simulink model "odom_waypoint"  (R2022a)
settings: Solver=FixedStepDiscrete  StartTime=0.0  StopTime=inf  FixedStep=0.05  RelTol=1e-3  EnableMultiTasking=on
undefined symbols (not defined in the file): Angular, Linear
libraries: robotlib x4
settings Model: Creator=The MathWorks, Inc.  LastModifiedBy=lcrist
settings SolverCC: AlgebraicLoopSolver=TrustRegion
settings DataIOCC: LimitDataPoints=on  SaveFormat=Array  ReturnWorkspaceOutputs=off
settings OptimizationCC: DefaultUnderspecifiedDataType=single  ZeroExternalMemoryAtStartup=off  ZeroInternalMemoryAtStartup=off  LifeSpan=1  MaxStackSize=64
settings DebuggingCC: SolverPrmCheckMsg=warning  UnconnectedInputMsg=warning  UnconnectedOutputMsg=warning  UnconnectedLineMsg=warning  SFUnexpectedBacktrackingDiag=warning  SFNoUnconditionalDefaultTransitionDiag=warning  SFExecutionAtInitializationDiag=none  SFMachineParentedDataDiag=warning  ArithmeticOperatorsInVariantConditions=warning
settings HardwareCC: ProdBitPerPointer=32  ProdBitPerSizeT=32  ProdBitPerPtrDiffT=32  ProdLargestAtomicFloat=None  ProdIntDivRoundTo=Undefined  ProdEndianess=Unspecified  ProdWordSize=32  ProdHWDeviceType=Generic->Unspecified (assume 32-bit Generic)  TargetHWDeviceType=Generic->Unspecified (assume 32-bit Generic)  UseEmbeddedCoderFeatures=off
settings ModelReferenceCC: PropagateSignalLabelsOutOfModel=off
settings SFSimCC: SimUseLocalCustomCode=off  CustomCodeUndefinedFunction=UseInterfaceOnly  SimTargetLang=C++
settings RTWCC: SystemTargetFile=ert.tlc  HardwareBoard=Robot Operating System (ROS)  TLCOptions=-aInlineSetEventsForThisBaseRateFcn=TLC_FALSE -aSuppressMultiTaskScheduler=TLC_FALSE -aRateBasedStepFcn=0  TemplateMakefile=ert_default_tmf  RTWUseLocalCustomCode=off  Toolchain=Catkin  TargetLang=C++
settings CodeAppCC: StateflowObjectComments=on
settings ERTTargetCC: MultiwordLength=2048  ERTCustomFileBanners=off  CodeInterfacePackaging=C++ class  SupportContinuousTime=on  SupportNonInlinedSFcns=on  RemoveResetFunc=off  SupportVariableSizeSignals=on  ModelStepFunctionPrototypeControlCompliant=off  RootIOFormat=Structure reference  ConvertIfToSwitch=off  SuppressUnreachableDefaultCases=off
settings ConfigComp: CovMetricSettings=dw  CovSaveCumulativeToWorkspaceVar=on  CovSaveSingleToWorkspaceVar=on  CovExternalEMLEnable=off  CovSFcnEnable=off

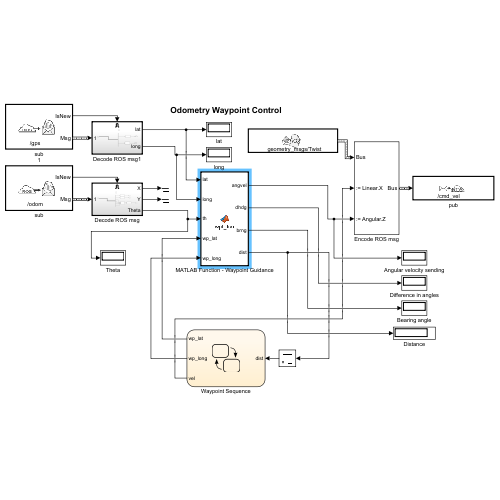
[thumbnail: Simulink's stored preview of the top-level diagram]
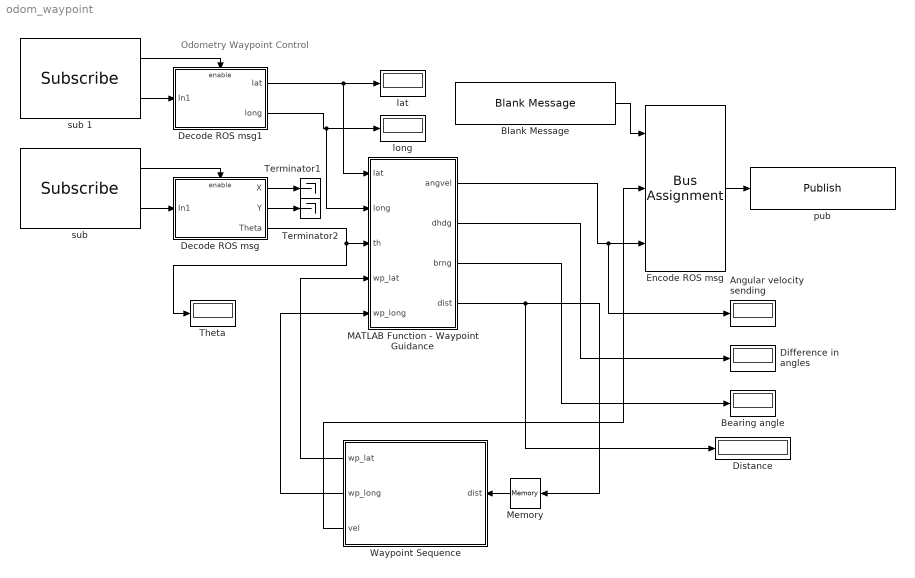
== system odom_waypoint ==
  note: Odometry Waypoint Control
  Angular velocity sending : Display
  Bearing angle : Display
  Blank Message : robotlib/Blank Message  messageClass=Message  entityType=geometry_msgs/Twist  messageType=geometry_msgs/Twist  SampleTime=inf  legacyBusStruct=off
  Decode ROS msg : Subsystem
  Decode ROS msg1 : Subsystem
  Difference in angles : Display
  Distance : Display
  Encode ROS msg : BusAssignment  AssignedSignals=Linear.X,Angular.Z
  MATLAB Function - Waypoint Guidance : MATLAB Function  TreatAsAtomicUnit=on
  Memory : Memory  InitialCondition=1
  Terminator1 : Terminator
  Terminator2 : Terminator
  Theta : Display
  Waypoint Sequence : Stateflow chart  TreatAsAtomicUnit=on
  lat : Display
  long : Display
  pub : robotlib/Publish  topicSource=Specify your own  topic=/cmd_vel  messageType=geometry_msgs/Twist  legacyBusStruct=off  messageQueueLength=105
  "sub " : robotlib/Subscribe  topicSource=Specify your own  topic=/odom  messageType=nav_msgs/Odometry  SampleTime=-1  legacyBusStruct=off  messageQueueLength=51
  sub 1 : robotlib/Subscribe  topicSource=Specify your own  topic=/gps  messageType=sensor_msgs/NavSatFix  SampleTime=-1  legacyBusStruct=off  messageQueueLength=51
  wires:
  Encode ROS msg/1 -> pub/1
  "sub "/1 -> Decode ROS msg/Enable
  "sub "/2 -> Decode ROS msg/1(In1)
  Blank Message/1 -> Encode ROS msg/1
  Decode ROS msg/3(Theta) -> MATLAB Function - Waypoint Guidance/3(th), Theta/1
  MATLAB Function - Waypoint Guidance/1(angvel) -> Encode ROS msg/3, Angular velocity sending/1
  Waypoint Sequence/1(wp_lat) -> MATLAB Function - Waypoint Guidance/4(wp_lat)
  Waypoint Sequence/2(wp_long) -> MATLAB Function - Waypoint Guidance/5(wp_long)
  Memory/1 -> Waypoint Sequence/1(dist)
  sub 1/2 -> Decode ROS msg1/1(In1)
  sub 1/1 -> Decode ROS msg1/Enable
  Decode ROS msg/1(X) -> Terminator1/1
  Decode ROS msg/2(Y) -> Terminator2/1
  Decode ROS msg1/1(lat) -> MATLAB Function - Waypoint Guidance/1(lat), lat/1
  Decode ROS msg1/2(long) -> MATLAB Function - Waypoint Guidance/2(long), long/1
  MATLAB Function - Waypoint Guidance/2(dhdg) -> Difference in angles/1
  MATLAB Function - Waypoint Guidance/3(brng) -> Bearing angle/1
  MATLAB Function - Waypoint Guidance/4(dist) -> Memory/1, Distance/1
  Waypoint Sequence/3(vel) -> Encode ROS msg/2

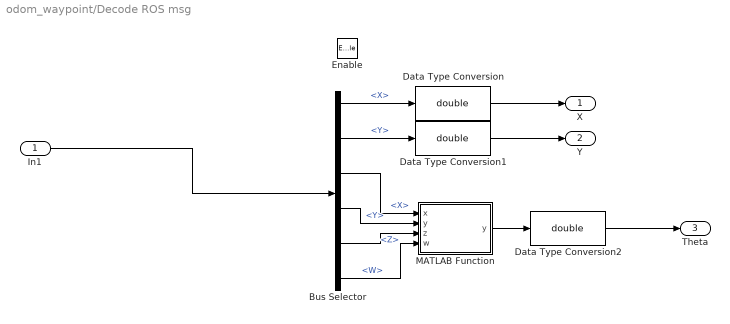
== system odom_waypoint/Decode ROS msg ==
  In1 : Inport
  Enable : EnablePort
  Bus Selector : BusSelector  DialogController=Simulink.DDGSource_BusSelector  OutputSignals=Pose.Pose.Position.X,Pose.Pose.Position.Y,Pose.Pose.Orientation.X,Pose.Pose.Orientation.Y,Pose.Pose.Orientation.Z,Pose.Pose.Orientation.W
  Data Type Conversion : DataTypeConversion  OutDataTypeStr=double  SaturateOnIntegerOverflow=off  RndMeth=Floor
  Data Type Conversion1 : DataTypeConversion  OutDataTypeStr=double  SaturateOnIntegerOverflow=off  RndMeth=Floor
  Data Type Conversion2 : DataTypeConversion  OutDataTypeStr=double  SaturateOnIntegerOverflow=off  RndMeth=Floor
  MATLAB Function : MATLAB Function  TreatAsAtomicUnit=on
  X : Outport  VectorParamsAs1DForOutWhenUnconnected=off
  Y : Outport  Port=2  VectorParamsAs1DForOutWhenUnconnected=off
  Theta : Outport  Port=3  VectorParamsAs1DForOutWhenUnconnected=off
  wires:
  In1/1 -> Bus Selector/1
  Bus Selector/2 -> Data Type Conversion1/1  "<Y>"
  Bus Selector/1 -> Data Type Conversion/1  "<X>"
  Data Type Conversion/1 -> X/1
  Data Type Conversion1/1 -> Y/1
  Data Type Conversion2/1 -> Theta/1
  MATLAB Function/1(y) -> Data Type Conversion2/1
  Bus Selector/3 -> MATLAB Function/1(x)  "<X>"
  Bus Selector/4 -> MATLAB Function/2("y ")  "<Y>"
  Bus Selector/5 -> MATLAB Function/3(z)  "<Z>"
  Bus Selector/6 -> MATLAB Function/4(w)  "<W>"

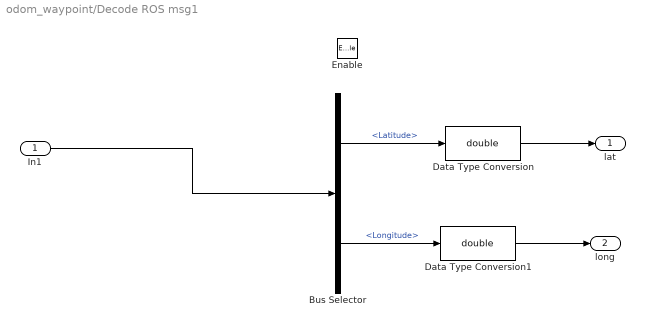
== system odom_waypoint/Decode ROS msg1 ==
  In1 : Inport
  Enable : EnablePort
  Bus Selector : BusSelector  DialogController=Simulink.DDGSource_BusSelector  OutputSignals=Latitude,Longitude
  Data Type Conversion : DataTypeConversion  OutDataTypeStr=double  SaturateOnIntegerOverflow=off  RndMeth=Floor
  Data Type Conversion1 : DataTypeConversion  OutDataTypeStr=double  SaturateOnIntegerOverflow=off  RndMeth=Floor
  lat : Outport  VectorParamsAs1DForOutWhenUnconnected=off
  long : Outport  Port=2  VectorParamsAs1DForOutWhenUnconnected=off
  wires:
  In1/1 -> Bus Selector/1
  Bus Selector/2 -> Data Type Conversion1/1  "<Longitude>"
  Bus Selector/1 -> Data Type Conversion/1  "<Latitude>"
  Data Type Conversion/1 -> lat/1
  Data Type Conversion1/1 -> long/1

== matlab function odom_waypoint/Decode ROS msg/MATLAB Function ==
  data: x input; y output; y input; z input; w input
function y = fcn(x,y,z,w)

eulZYX = quat2eul([x,y,z,w]);

y = eulZYX(3);

== matlab function odom_waypoint/MATLAB Function - Waypoint Guidance ==
  data: angvel output; lat input; long input; th input; wp_lat input; wp_long input; dhdg output; brng output; dist output
function [angvel, dhdg, brng, dist]  = wpt_fcn(lat,long,th,wp_lat,wp_long)
% Function to implement waypoint guidance
% Inputs:
%  - lat: Current lattitude position
%  - long: Current longitude position
%  - th: Current theta position
%  - wp_lat: Current waypoint goals, lattitude
%  - wp_long: Current waypoint goals, longitude
% Outputs:
%  - dist: Distance from current position to current waypoint goal
%  - angvel: Desired angular velocity [rad/s, clockwise]
%  - linvel: Desired linear velocity

R = 6371e3;
lat_i = lat*(pi/180);
lat_f = wp_lat*(pi/180);
long_i = long*(pi/180);
long_f = wp_long*(pi/180);
dlat = (wp_lat-lat)*(pi/180);
dlong = (wp_long-long)*(pi/180);

a = sin(dlat/2)*sin(dlat/2) + cos(lat_i)*cos(lat_f)*sin(dlong/2)*sin(dlong/2);

c = 2*atan2(sqrt(a), sqrt(1-a));

d = R*c;

% Angle from current location to waypoint
y = sin(long_f-long_i)*cos(lat_f);
x = (cos(lat_i)*sin(lat_f)) - (sin(lat_i)*cos(lat_f)*cos(long_f-long_i));
th2 = atan2(y,x);
brng = mod((th2*(180/pi))+360, 360);

% Convert theta, from odom, to radians and set north to 90 degrees
th = th * (180/pi);
th = th - 90;

%Unwrap angle
while th < -180
    th = th + 360;
end
while th > 180
    th = th - 360;
end

while brng < -180
    brng = brng + 360;
end
while brng > 180
    brng = brng - 360;
end

% Difference (error) between current turtle angle and desired angle
dhdg = th - brng;


% while dhdg < -180
%     dhdg = dhdg + 360;
% end
% while dhdg > 180
%     dhdg = dhdg - 360;
% end

% Proportional Control
% Gains
Kphdg = 1.5;  % Proportional gain for heading

% Specify commands to turtle
angvel=Kphdg*dhdg*(pi/180);
dist = d;

end

== stateflow chart odom_waypoint/Waypoint Sequence ==
  settings: executeAtInitialization=1
  state Waypoint9
    entry: wp_lat=42.47485356052358;
    wp_long=-83.24884397403449;
  state Waypoint5
    entry: wp_lat=42.475261492954594;
    wp_long=-83.24889664565237;
  state Waypoint1
    entry: wp_lat=42.47517731432692;
    wp_long=-83.2484420897516; vel = 1;
  state Waypoint6
    entry: wp_lat=42.47520033920633;
    wp_long=-83.24894249178445;
  state Waypoint10
    entry: wp_lat=42.47485140097793;
    wp_long=-83.24857377780822;
  state Waypoint7
    entry: wp_lat=42.474955004259336;
    wp_long=-83.24893956650178;
  state Waypoint11
    entry: wp_lat=42.47486722843812;
    wp_long=-83.24847233210649;
  state Waypoint2
    entry: wp_lat=42.47524638239457;
    wp_long=-83.24846745042454;
  state Waypoint3
    entry: wp_lat=42.47528379470202;
    wp_long=-83.24855523999123;
  state Waypoint12
    entry: wp_lat=42.47495572150004;
    wp_long=-83.24844379946735; vel = 0;
  state Waypoint8
    entry: wp_lat=42.474882339044214;
    wp_long=-83.24892688612681;
  state Waypoint4
    entry: wp_lat=42.47528451527216;
    wp_long=-83.24879227301304;
  Waypoint4 -> Waypoint5 : [dist<0.5]
  Waypoint8 -> Waypoint9 : [dist<0.5]
  Waypoint9 -> Waypoint10 : [dist<0.5]
  Waypoint5 -> Waypoint6 : [dist<0.5]
  (default) -> Waypoint1
  Waypoint6 -> Waypoint7 : [dist<0.5]
  Waypoint10 -> Waypoint11 : [dist<0.5]
  Waypoint1 -> Waypoint2 : [dist<0.5]
  Waypoint7 -> Waypoint8 : [dist<0.5]
  Waypoint11 -> Waypoint12 : [dist<0.5]
  Waypoint2 -> Waypoint3 : [dist<0.5]
  Waypoint3 -> Waypoint4 : [dist<0.5]
  data: dist input double; wp_lat output double; wp_long output double; vel output
